simulink library "libMdl_TrainEndDataGenerator"  (R2018a)
settings: Solver=VariableStepAuto  StartTime=0.0  StopTime=10.0  RelTol=1e-3
settings Model: Creator=hwinter  LastModifiedBy=Hanno

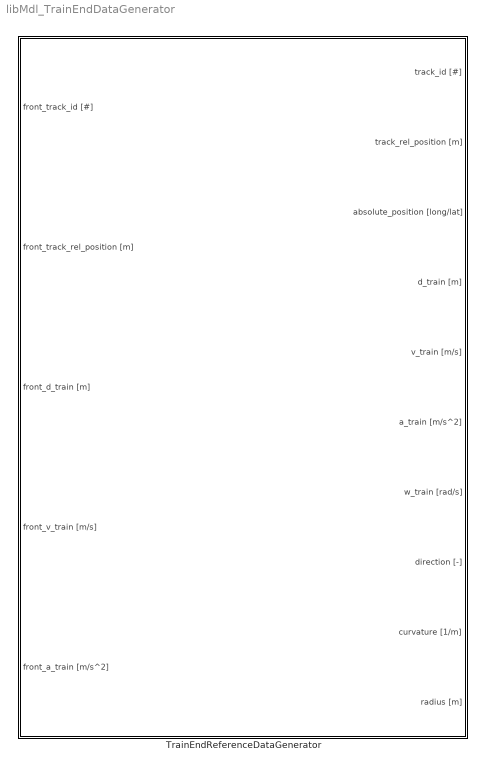
== system libMdl_TrainEndDataGenerator ==
  TrainEndReferenceDataGenerator : Subsystem  TreatAsAtomicUnit=on  mask(Reference Data Generator (train end)){mv_train_length=[], mv_track_map=[], mv_track_map_rot_angle=[]}
      mask prompts: mv_train_length "Train length:"; mv_track_map "Track Map:"; mv_track_map_rot_angle "Track Map Rotation Angle:"
      mask help:
      | Train length:
      | Length of the train in meters
      |
      | Track Map:
      | Track-Map in matrix format
      | (for more details see: Track Generator Tool)
      |
      | Track Map Rotation Angle:
      | Initial alignment of the Track-Map in degrees
      mask Display:
      | str1 = sprintf('\\color{black}{\\bfReference Data Generator (train end)}\n\n');
      | str2 = sprintf('Sample Time: %0.2f\n\n',-1);
      | str3 = sprintf('Train length [m]: %3.0f\n\n',mv_train_length);
      | if length(mv_track_map) == 1
      |     str4 = sprintf('Map: %0.2f\n',mv_track_map);
      | else
      |     str4 = sprintf('Map: [...]\n');
      | end % if
      | str5 = sprintf('\\phi_{Map}: %5.1f',mv_track_map_rot_angle);
      | str = [str1,str2,str3,str4,str5];
      | 
      | text( 0.5,0.5, ...
      |       str, ...
      |       'horizontalAlignment', 'center', ...
      |       'texmode','on' ...
      |     )

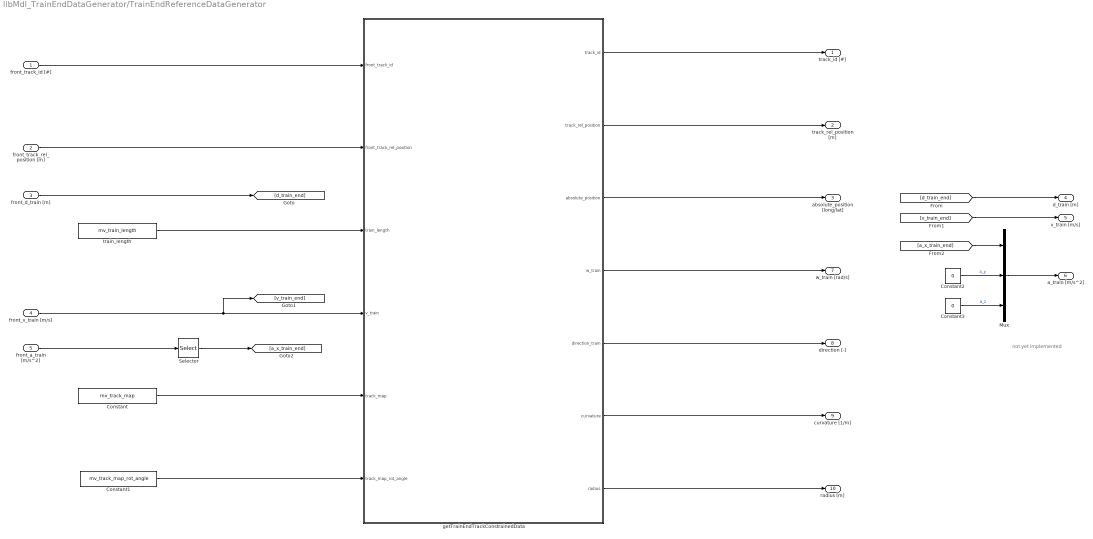
== system libMdl_TrainEndDataGenerator/TrainEndReferenceDataGenerator ==
  note: not yet implemented
  front_track_id [#] : Inport
  front_track_rel_position [m] : Inport  Port=2
  front_d_train [m] : Inport  Port=3
  front_v_train [m/s] : Inport  Port=4
  front_a_train [m/s^2] : Inport  Port=5
  Constant : Constant  Value=mv_track_map  VectorParams1D=off
  Constant1 : Constant  Value=mv_track_map_rot_angle
  Constant2 : Constant  Value=0
  Constant3 : Constant  Value=0
  Mux : Mux  Inputs=3
  Selector : Selector  InputPortWidth=3  IndexOptions=Index vector (dialog)  Indices=1  OutputSizes=1
  getTrainEndTrackConstrainedData : MATLAB Function  TreatAsAtomicUnit=on
  train_length : Constant  Value=mv_train_length  VectorParams1D=off
  track_id [#] : Outport
  track_rel_position [m] : Outport  Port=2
  absolute_position [long/lat] : Outport  Port=3
  d_train [m] : Outport  Port=4
  v_train [m/s] : Outport  Port=5
  a_train [m/s^2] : Outport  Port=6
  w_train [rad/s] : Outport  Port=7
  direction [-] : Outport  Port=8
  curvature [1/m] : Outport  Port=9
  radius [m] : Outport  Port=10
  wires:
  train_length/1 -> getTrainEndTrackConstrainedData/3(train_length)
  Selector/1 -> [a_x_train_end]
  Constant/1 -> getTrainEndTrackConstrainedData/5(track_map)
  Mux/1 -> a_train [m/s^2]/1
  [a_x_train_end] -> Mux/1
  Constant3/1 -> Mux/3  "a_z"
  Constant2/1 -> Mux/2  "a_y"
  [v_train_end] -> v_train [m/s]/1
  [d_train_end] -> d_train [m]/1
  front_a_train [m/s^2]/1 -> Selector/1
  front_d_train [m]/1 -> [d_train_end]
  front_v_train [m/s]/1 -> getTrainEndTrackConstrainedData/4(v_train), [v_train_end]
  getTrainEndTrackConstrainedData/2(track_rel_position) -> track_rel_position [m]/1
  getTrainEndTrackConstrainedData/7(radius) -> radius [m]/1
  getTrainEndTrackConstrainedData/6(curvature) -> curvature [1/m]/1
  getTrainEndTrackConstrainedData/5(direction_train) -> direction [-]/1
  getTrainEndTrackConstrainedData/4(w_train) -> w_train [rad/s]/1
  getTrainEndTrackConstrainedData/3(absolute_position) -> absolute_position [long/lat]/1
  getTrainEndTrackConstrainedData/1(track_id) -> track_id [#]/1
  front_track_id [#]/1 -> getTrainEndTrackConstrainedData/1(front_track_id)
  front_track_rel_position [m]/1 -> getTrainEndTrackConstrainedData/2(front_track_rel_position)
  Constant1/1 -> getTrainEndTrackConstrainedData/6(track_map_rot_angle)

== matlab function libMdl_TrainEndDataGenerator/TrainEndReferenceDataGenerator/getTrainEndTrackConstrainedData ==
  data: front_track_id input; front_track_rel_position input; train_length input; v_train input; track_id output; track_rel_position output; absolute_position output; w_train output; direction_train output; track_map input; curvature output; track_map_rot_angle input; radius output
function [track_id,track_rel_position,absolute_position,w_train,direction_train,curvature,radius] = simFcn_getTrainEndTrackConstrainedData(front_track_id,front_track_rel_position,train_length,v_train,track_map,track_map_rot_angle)

% Init ____________________________________________________________________

coder.extrinsic('calcTrackProperties','getTrackAbsPosition','getTrackRelPosition');

track_id = coder.nullcopy(zeros(1,1));
track_rel_position = coder.nullcopy(zeros(1,1));
absolute_position = coder.nullcopy(zeros(2,1));
w_train = coder.nullcopy(zeros(3,1));
direction_train = coder.nullcopy(zeros(2,1));
curvature = coder.nullcopy(zeros(1,1));
radius = coder.nullcopy(zeros(1,1));
front_abs_position = coder.nullcopy(zeros(1,1));
end_track_id = coder.nullcopy(zeros(1,1));
end_rel_position = coder.nullcopy(zeros(1,1));

% Calculations ____________________________________________________________

% Calculate relative train end position
front_abs_position = getTrackAbsPosition(front_track_id,front_track_rel_position,track_map);
end_abs_position = front_abs_position - train_length;
[end_track_id,end_rel_position,~] = getTrackRelPosition(end_abs_position,track_map);

% set direction of train on the track
track_direction = sign(v_train);
track_direction(track_direction==0) = 1;

% calculate output values
[track_id,track_rel_position,~,absolute_position,direction_train,curvature,radius,~] = calcTrackProperties(0,end_track_id,end_rel_position,track_map,track_map_rot_angle,track_direction);

w_train = [0;0;-1*curvature*v_train]; % roll rate not implemented yet 
                                      % pitch rate not implemented yet
                                      % yaw rate: multiply by minus 1 to transform from track coordinates (curvature) to train coordinates (turn rate)
 
end % function
